simulink model "skipperLQI"  (R2024a)
settings: Solver=ode113  StartTime=0.0  StopTime=10  RelTol=1e-3
libraries: matrix_library x2
settings Model: Creator=nehir  LastModifiedBy=nehir

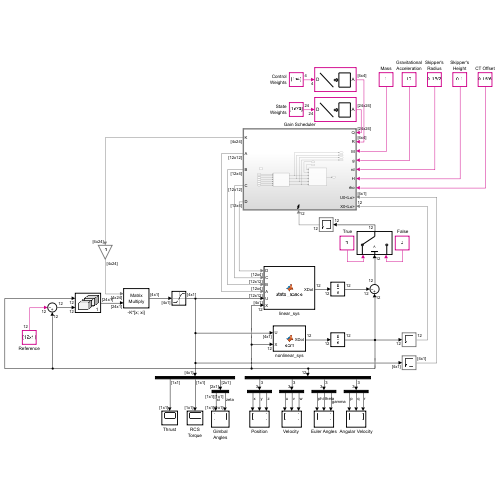
[thumbnail: Simulink's stored preview of the top-level diagram]
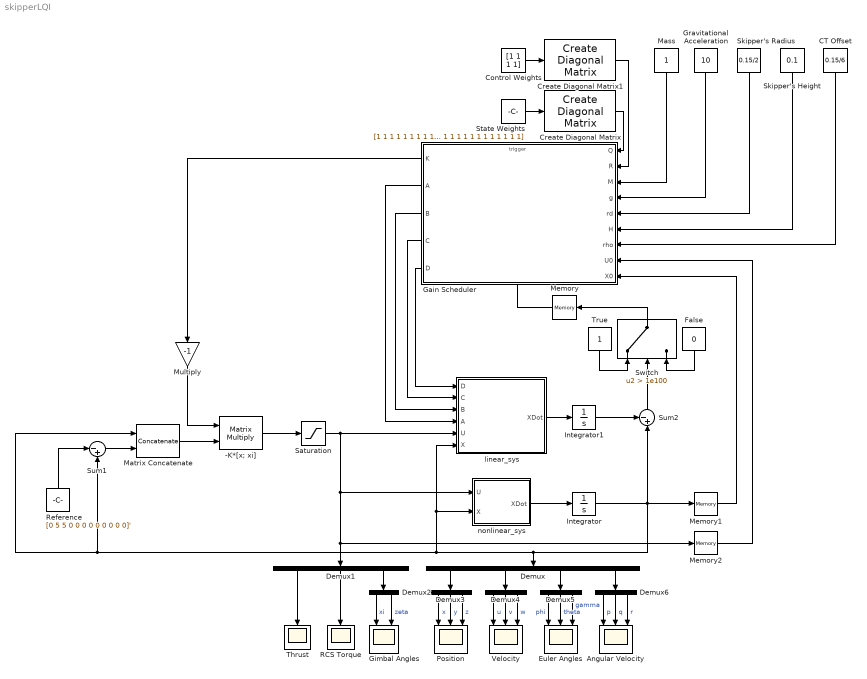
== system skipperLQI ==
  " False" : Constant  Value=0
  " True" : Constant
  -K*[x; xi] : Product  Multiplication=Matrix(*)
  Angular Velocity : Scope  NumInputPorts=3
  CT Offset : Constant  Value=0.15/6
  Control Weights : Constant  Value=[1 1 1 1]
  Create Diagonal Matrix : matrix_library/Create Diagonal Matrix
      settings: LibrarySourceBlock=|
      | simulink/Matrix
      | Operations/Create Diagonal
      | Matrix
  Create Diagonal Matrix1 : matrix_library/Create Diagonal Matrix
      settings: LibrarySourceBlock=|
      | simulink/Matrix
      | Operations/Create Diagonal
      | Matrix
  Demux : Demux  Outputs=[3 3 3 3]
  Demux1 : Demux  Outputs=[1 1 2]
  Demux2 : Demux  Outputs=[1 1]
  Demux{3..6} (4 alike) : Demux  Outputs=[1 1 1]
  Euler Angles : Scope  NumInputPorts=3
  Gain Scheduler : Subsystem  TreatAsAtomicUnit=on
  Gimbal Angles : Scope  NumInputPorts=2
  Gravitational Acceleration : Constant  Value=10
  Integrator : Integrator  InitialCondition=[0 0 0 0 0 0 0 0 0 0 0 0]'
  Integrator1 : Integrator  InitialCondition=[0 0 0 0 0 0 0 0 0 0 0 0]'
  Mass : Constant
  Matrix Concatenate : Concatenate  Mode=Multidimensional array
  Memory : Memory  InitialCondition=1
  Memory1 : Memory  InitialCondition=[0 0 0 0 0 0 0 0 0 0 0 0]'
  Memory2 : Memory  InitialCondition=[10 1 -pi/36 pi/36]'
  Multiply : Gain  Gain=-1
  Position : Scope  NumInputPorts=3
  RCS Torque : Scope
  Reference : Constant  Value=[0 5 5 0 0 0 0 0 0 0 0 0]'
  Saturation : Saturate  UpperLimit=[15 1 pi/18 pi/18]'  LowerLimit=[0 -1 -pi/18 -pi/18]'
  Skipper's Height : Constant  Value=0.1
  Skipper's Radius : Constant  Value=0.15/2
  State Weights : Constant  Value=[1 1 1 1 1 1 1 1 1 1 1 1 1 1 1 1 1 1 1 1 1 1 1 1]
  Sum1 : Sum  Inputs=|-+
  Sum2 : Sum  Inputs=-+|
  Switch : Switch  Criteria=u2 > Threshold  Threshold=1e100  ZeroCross=off  SaturateOnIntegerOverflow=off  InputSameDT=off
  Thrust : Scope
  "Velocity " : Scope  NumInputPorts=3
  linear_sys : MATLAB Function  TreatAsAtomicUnit=on
  nonlinear_sys : MATLAB Function  TreatAsAtomicUnit=on
  wires:
  Demux1/2 -> RCS Torque/1
  Demux1/1 -> Thrust/1
  Demux/1 -> Demux3/1
  Demux/2 -> Demux4/1
  Demux/3 -> Demux5/1
  Demux/4 -> Demux6/1
  Demux1/3 -> Demux2/1
  Demux2/1 -> Gimbal Angles/1  "xi"
  Demux2/2 -> Gimbal Angles/2  "zeta"
  Demux3/1 -> Position/1  "x"
  Demux3/3 -> Position/3  "z"
  Demux4/1 -> "Velocity "/1  "u"
  Demux4/2 -> "Velocity "/2  "v"
  Demux4/3 -> "Velocity "/3  "w"
  Demux5/1 -> Euler Angles/1  "phi"
  Demux5/2 -> Euler Angles/2  "theta"
  Demux5/3 -> Euler Angles/3  "gamma"
  Demux3/2 -> Position/2  "y"
  Demux6/1 -> Angular Velocity/1  "p"
  Demux6/2 -> Angular Velocity/2  "q"
  Demux6/3 -> Angular Velocity/3  "r"
  nonlinear_sys/1(XDot) -> Integrator/1
  -K*[x; xi]/1 -> Saturation/1
  Reference/1 -> Sum1/1
  Sum2/1 -> Switch/2
  linear_sys/1(XDot) -> Integrator1/1
  Integrator1/1 -> Sum2/1
  State Weights/1 -> Create Diagonal Matrix/1
  Control Weights/1 -> Create Diagonal Matrix1/1
  Multiply/1 -> -K*[x; xi]/1
  Gain Scheduler/3(B) -> linear_sys/3(B)
  Gain Scheduler/1(K) -> Multiply/1
  Switch/1 -> Memory/1
  " True"/1 -> Switch/1
  " False"/1 -> Switch/3
  Create Diagonal Matrix/1 -> Gain Scheduler/1(Q)
  Create Diagonal Matrix1/1 -> Gain Scheduler/2(R)
  Mass/1 -> Gain Scheduler/3(M)
  Gravitational Acceleration/1 -> Gain Scheduler/4(g)
  Skipper's Radius/1 -> Gain Scheduler/5(rd)
  Skipper's Height/1 -> Gain Scheduler/6(H)
  CT Offset/1 -> Gain Scheduler/7(rho)
  Gain Scheduler/5(D) -> linear_sys/1(D)
  Gain Scheduler/4(C) -> linear_sys/2(C)
  Gain Scheduler/2(A) -> linear_sys/4(A)
  Integrator/1 -> Memory1/1, Sum2/2, Matrix Concatenate/1, Sum1/2, nonlinear_sys/2(X), linear_sys/6(X), Demux/1
  Memory2/1 -> Gain Scheduler/8(U0)
  Memory1/1 -> Gain Scheduler/9(X0)
  Memory/1 -> Gain Scheduler/Trigger
  Saturation/1 -> Demux1/1, Memory2/1, nonlinear_sys/1(U), linear_sys/5(U)
  Sum1/1 -> Matrix Concatenate/2
  Matrix Concatenate/1 -> -K*[x; xi]/2

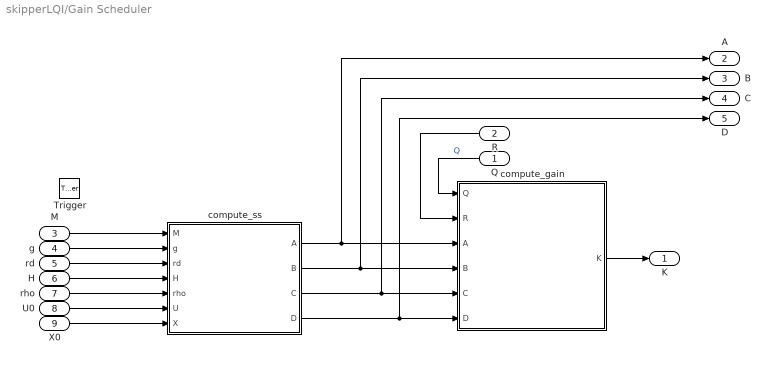
== system skipperLQI/Gain Scheduler ==
  Q : Inport
  R : Inport  Port=2
  M : Inport  Port=3
  g : Inport  Port=4
  rd : Inport  Port=5
  H : Inport  Port=6
  rho : Inport  Port=7
  U0 : Inport  Port=8  LatchByDelayingOutsideSignal=on
  X0 : Inport  Port=9  LatchByDelayingOutsideSignal=on
  Trigger : TriggerPort  VariantControl=(inherit)  ZeroCross=off  InitialTriggerSignalState=negative
  compute_gain : MATLAB Function  TreatAsAtomicUnit=on
  compute_ss : MATLAB Function  TreatAsAtomicUnit=on
  K : Outport
  A : Outport  Port=2
  B : Outport  Port=3
  C : Outport  Port=4
  D : Outport  Port=5
  wires:
  M/1 -> compute_ss/1(M)
  R/1 -> compute_gain/2(R)
  Q/1 -> compute_gain/1(Q)  "Q"
  U0/1 -> compute_ss/6(U)
  rho/1 -> compute_ss/5(rho)
  H/1 -> compute_ss/4(H)
  rd/1 -> compute_ss/3(rd)
  g/1 -> compute_ss/2(g)
  X0/1 -> compute_ss/7(X)
  compute_gain/1(K) -> K/1
  compute_ss/1(A) -> A/1, compute_gain/3(A)
  compute_ss/2(B) -> B/1, compute_gain/4(B)
  compute_ss/3(C) -> C/1, compute_gain/5(C)
  compute_ss/4(D) -> D/1, compute_gain/6(D)

== matlab function skipperLQI/Gain Scheduler/compute_ss ==
  data: M input; g input; rd input; H input; rho input; U input; X input; A output; B output; C output; D output
function [A, B, C, D] = compute_ss(M, g, rd, H, rho, U, X)
% ________________________________________________________________________
%
%                           STATE SPACE MATRICES
% ________________________________________________________________________
% 
% BY:       FLORIDA ROCKET LAB - GNC SUBTEAM
% EDITORS:  N. HIRSCH, L. DAPP
% DATE:     1/20/25
%
% OVERVIEW: Calculates A, B, C, D, matices for use in a state
% space Simulink model and LQR controller as well as the disturbance, d.

    save('basepoints.mat', 'U', 'X')
    % Calculate rotational inertias in body frame.
    Ixx = M*rd^2/2;
    Iyy = M*(3*rd^2+H^2)/12;
    Izz = Iyy;
    
    % Initialize state space matricies. Since they are sparse simply use zeros
    % and then input non-zero terms individually.
    % x = [x y z u v w phi theta psi p q r]
    % u = [T tauR xi zeta]
    x0 = X(1);
    y0 = X(2);
    z0 = X(3);
    u0 = X(4);
    v0 = X(5);
    w0 = X(6);
    phi0 = X(7);
    theta0 = X(8);
    psi0 = X(9);
    p0 = X(10);
    q0 = X(11);
    r0 = X(12);

    T0 = U(1);
    tauR0 = U(2);
    xi0 = U(3);
    zeta0 = U(4);

    % BEGIN "A"; Do not modify this. The python script looks for this line.
    A = [
        0 0 0 cos(psi0)*cos(theta0) sin(phi0)*sin(theta0)*cos(psi0)-sin(psi0)*cos(phi0) sin(phi0)*sin(psi0)+sin(theta0)*cos(phi0)*cos(psi0) v0*sin(phi0)*sin(psi0)+v0*sin(theta0)*cos(phi0)*cos(psi0)-w0*sin(phi0)*sin(theta0)*cos(psi0)+w0*sin(psi0)*cos(phi0) -u0*sin(theta0)*cos(psi0)+v0*sin(phi0)*cos(psi0)*cos(theta0)+w0*cos(phi0)*cos(psi0)*cos(theta0) -u0*sin(psi0)*cos(theta0)-v0*sin(phi0)*sin(psi0)*sin(theta0)-v0*cos(phi0)*cos(psi0)+w0*sin(phi0)*cos(psi0)-w0*sin(psi0)*sin(theta0)*cos(phi0) 0 0 0;
        0 0 0 sin(psi0)*cos(theta0) sin(phi0)*sin(psi0)*sin(theta0)+cos(phi0)*cos(psi0) -sin(phi0)*cos(psi0)+sin(psi0)*sin(theta0)*cos(phi0) -v0*sin(phi0)*cos(psi0)+v0*sin(psi0)*sin(theta0)*cos(phi0)-w0*sin(phi0)*sin(psi0)*sin(theta0)-w0*cos(phi0)*cos(psi0) -u0*sin(psi0)*sin(theta0)+v0*sin(phi0)*sin(psi0)*cos(theta0)+w0*sin(psi0)*cos(phi0)*cos(theta0) u0*cos(psi0)*cos(theta0)+v0*sin(phi0)*sin(theta0)*cos(psi0)-v0*sin(psi0)*cos(phi0)+w0*sin(phi0)*sin(psi0)+w0*sin(theta0)*cos(phi0)*cos(psi0) 0 0 0;
        0 0 0 -sin(theta0) sin(phi0)*cos(theta0) cos(phi0)*cos(theta0) v0*cos(phi0)*cos(theta0)-w0*sin(phi0)*cos(theta0) -u0*cos(theta0)-v0*sin(phi0)*sin(theta0)-w0*sin(theta0)*cos(phi0) 0 0 0 0;
        0 0 0 0 r0 -q0 0 g*sin(theta0)*cos(psi0) g*sin(psi0)*cos(theta0) 0 -w0 v0;
        0 0 0 -r0 0 p0 -g*sin(phi0)*sin(psi0)-g*sin(theta0)*cos(phi0)*cos(psi0) -g*sin(phi0)*cos(psi0)*cos(theta0) g*sin(phi0)*sin(psi0)*sin(theta0)+g*cos(phi0)*cos(psi0) w0 0 -u0;
        0 0 0 q0 -p0 0 g*sin(phi0)*sin(theta0)*cos(psi0)-g*sin(psi0)*cos(phi0) -g*cos(phi0)*cos(psi0)*cos(theta0) -g*sin(phi0)*cos(psi0)+g*sin(psi0)*sin(theta0)*cos(phi0) -v0 u0 0;
        0 0 0 0 0 0 q0*cos(phi0)*tan(theta0)-r0*sin(phi0)*tan(theta0) q0*sin(phi0)*tan(theta0)^2+q0*sin(phi0)+r0*cos(phi0)*tan(theta0)^2+r0*cos(phi0) 0 1 sin(phi0)*tan(theta0) cos(phi0)*tan(theta0);
        0 0 0 0 0 0 -q0*sin(phi0)-r0*cos(phi0) 0 0 0 cos(phi0) -sin(phi0);
        0 0 0 0 0 0 q0*cos(phi0)/cos(theta0)-r0*sin(phi0)/cos(theta0) q0*sin(phi0)*sin(theta0)/cos(theta0)^2+r0*sin(theta0)*cos(phi0)/cos(theta0)^2 0 0 sin(phi0)/cos(theta0) cos(phi0)/cos(theta0);
        0 0 0 0 0 0 0 0 0 0 Iyy*r0/Ixx-Izz*r0/Ixx Iyy*q0/Ixx-Izz*q0/Ixx;
        0 0 0 0 0 0 0 0 0 -Ixx*r0/Iyy+Izz*r0/Iyy 0 -Ixx*p0/Iyy+Izz*p0/Iyy;
        0 0 0 0 0 0 0 0 0 Ixx*q0/Izz-Iyy*q0/Izz Ixx*p0/Izz-Iyy*p0/Izz 0;
    ];
    % END "A"; Do not modify this. The python script looks for this line.

    % u = [T tauR xi zeta]

    % BEGIN "B"; Do not modify this. The python script looks for this line.
    B = [
        0 0 0 0;
        0 0 0 0;
        0 0 0 0;
        cos(xi0)*cos(zeta0)/M 0 -T0*sin(xi0)*cos(zeta0)/M -T0*sin(zeta0)*cos(xi0)/M;
        sin(zeta0)/M 0 0 T0*cos(zeta0)/M;
        -sin(xi0)*cos(zeta0)/M 0 -T0*cos(xi0)*cos(zeta0)/M T0*sin(xi0)*sin(zeta0)/M;
        0 0 0 0;
        0 0 0 0;
        0 0 0 0;
        0 1/Ixx 0 0;
        -rho*sin(xi0)*cos(zeta0)/Iyy 0 -T0*rho*cos(xi0)*cos(zeta0)/Iyy T0*rho*sin(xi0)*sin(zeta0)/Iyy;
        -rho*sin(zeta0)/Izz 0 0 -T0*rho*cos(zeta0)/Izz;
    ];
    % END "B"; Do not modify this. The python script looks for this line.
   
    C = diag(ones(1, 12));
    
    D = zeros(size(B));
end

== matlab function skipperLQI/nonlinear_sys ==
  data: U input; XDot output; X input
function XDot = eom(U, X)
    R = 0.15/2; H = 0.1; g = 10; M = 1;
    rho2 = 0.15/6;
    Ixx = M*R^2/2;
    Iyy = M*(3*R^2+H^2)/12;
    Izz = Iyy;

    x = X(1);
    y = X(2);
    z = X(3);
    u = X(4);
    v = X(5);
    w = X(6);
    phi = X(7);
    theta = X(8);
    psi = X(9);
    p = X(10);
    q = X(11);
    r = X(12);

    T = U(1);
    tauR = U(2);
    xi = U(3);
    zeta = U(4);

    xDot = w*(sin(phi)*sin(psi) + cos(phi)*cos(psi)*sin(theta)) - v*(cos(phi)*sin(psi) - cos(psi)*sin(phi)*sin(theta)) + u*cos(psi)*cos(theta);
    yDot = v*(cos(phi)*cos(psi) + sin(phi)*sin(psi)*sin(theta)) - w*(cos(psi)*sin(phi) - cos(phi)*sin(psi)*sin(theta)) + u*cos(theta)*sin(psi);
    zDot = w*cos(phi)*cos(theta) - u*sin(theta) + v*cos(theta)*sin(phi);
    uDot = (T*cos(xi)*cos(zeta) - M*q*w + M*r*v - M*g*cos(psi)*cos(theta))/M;
    vDot = (T*sin(zeta) + M*p*w - M*r*u + M*g*cos(phi)*sin(psi) - M*g*cos(psi)*sin(phi)*sin(theta))/M;
    wDot = -(T*cos(zeta)*sin(xi) + M*p*v - M*q*u + M*g*sin(phi)*sin(psi) + M*g*cos(phi)*cos(psi)*sin(theta))/M;
    phiDot = p + r*cos(phi)*tan(theta) + q*sin(phi)*tan(theta);
    thetaDot = q*cos(phi) - r*sin(phi);
    psiDot = (r*cos(phi))/cos(theta) + (q*sin(phi))/cos(theta);
    pDot = (tauR + Iyy*q*r - Izz*q*r)/Ixx;
    qDot = -(Ixx*p*r - Izz*p*r + T*rho2*cos(zeta)*sin(xi))/Iyy;
    rDot = -(T*rho2*sin(zeta) - Ixx*p*q + Iyy*p*q)/Izz;

    XDot = [xDot yDot zDot uDot vDot wDot phiDot thetaDot psiDot pDot qDot rDot]';
end

== matlab function skipperLQI/linear_sys ==
  data: D input; C input; B input; A input; U input; XDot output; X input
function XDot = state_space(D, C, B, A, U, X)
    XDot = A*X + B*U;
end

== matlab function skipperLQI/Gain Scheduler/compute_gain ==
  data: Q input; R input; A input; K output; B input; C input; D input
function K = compute_gain(Q, R, A, B, C, D)

    % Declare 'lqr' as extrinsic so we can call it in simulation
    coder.extrinsic('lqi');
    coder.extrinsic('ss');
    save('matrices.mat', 'A', 'B', 'C', 'D', 'Q', 'R')

    sys = ss(A, B, C, D);
    K = zeros(4, 24);
    K = lqi(sys, Q, R);
end
